simulink model "lab_1_n_4"  (R2021b)
settings: Solver=VariableStepAuto  StartTime=0.0  StopTime=100.0  RelTol=1e-3
libraries: simulink x1
settings Model: Creator=peter  LastModifiedBy=peter

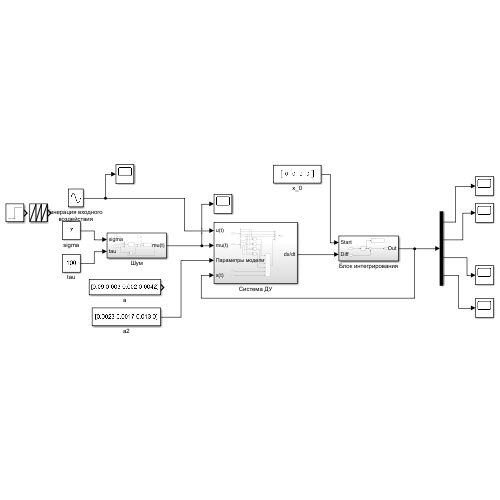
[thumbnail: Simulink's stored preview of the top-level diagram]
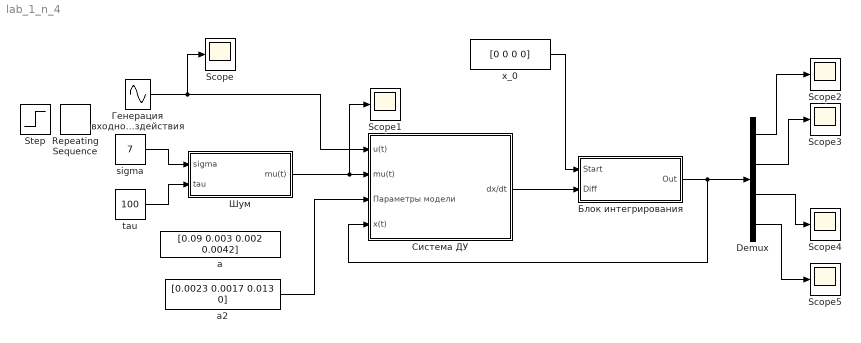
== system lab_1_n_4 ==
  Demux : Demux
  Repeating Sequence : simulink/Sources/Repeating Sequence  rep_seq_t=[0 2]  rep_seq_y=[0 2]
  Scope{,1..5} (6 alike) : Scope
  Step : Step  Time=10  SampleTime=0
  a : Constant  Value=[0.09 0.003 0.002 0.0042]
  a2 : Constant  Value=[0.0023 0.0017 0.013 0]
  sigma : Constant  Value=7
  tau : Constant  Value=100
  x_0 : Constant  Value=[0 0 0 0]
  Блок интегрирования : Subsystem
  Генерация входного воздействия : Sin  Frequency=0.05  SampleTime=0
  Система ДУ : Subsystem
  Шум : Subsystem
  wires:
  Demux/1 -> Scope2/1
  Demux/2 -> Scope3/1
  Demux/4 -> Scope5/1
  Demux/3 -> Scope4/1
  Блок интегрирования/1(Out) -> Система ДУ/4(x(t)), Demux/1
  x_0/1 -> Блок интегрирования/1(Start)
  Система ДУ/1(dx/dt) -> Блок интегрирования/2(Diff)
  Шум/1(mu(t)) -> Scope1/1, Система ДУ/2(mu(t))
  tau/1 -> Шум/2(tau)
  sigma/1 -> Шум/1(sigma)
  Генерация входного воздействия/1 -> Scope/1, Система ДУ/1(u(t))
  a2/1 -> Система ДУ/3(Параметры модели)

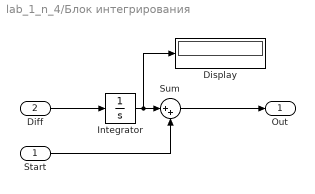
== system lab_1_n_4/Блок интегрирования ==
  Start : Inport
  Diff : Inport  Port=2
  Display : Display
  Integrator : Integrator
  Sum : Sum  Inputs=|++
  Out : Outport
  wires:
  Diff/1 -> Integrator/1
  Sum/1 -> Out/1
  Integrator/1 -> Display/1, Sum/1
  Start/1 -> Sum/2

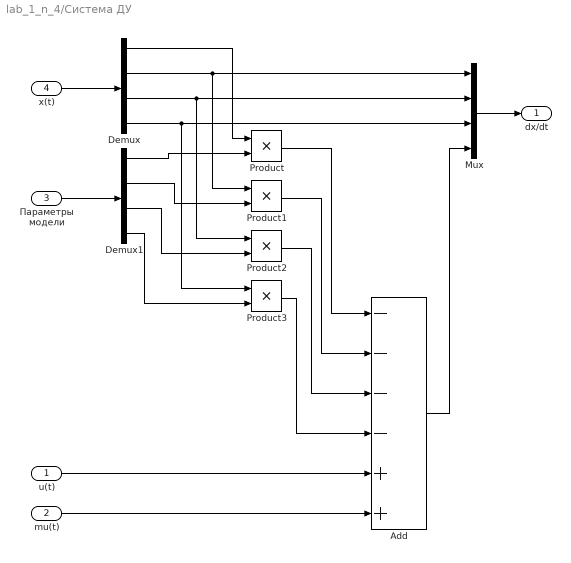
== system lab_1_n_4/Система ДУ ==
  u(t) : Inport
  mu(t) : Inport  Port=2
  Параметры модели : Inport  Port=3
  x(t) : Inport  Port=4
  Add : Sum  Inputs=----++
  Demux : Demux
  Demux1 : Demux
  Mux : Mux
  Product{,1..3} (4 alike) : Product
  dx/dt : Outport
  wires:
  x(t)/1 -> Demux/1
  Параметры модели/1 -> Demux1/1
  Mux/1 -> dx/dt/1
  Demux1/1 -> Product/2
  Demux1/2 -> Product1/2
  Demux1/3 -> Product2/2
  Demux/1 -> Product/1
  Demux/2 -> Product1/1, Mux/1
  Demux/3 -> Product2/1, Mux/2
  Product/1 -> Add/1
  Product1/1 -> Add/2
  Product2/1 -> Add/3
  Demux1/4 -> Product3/2
  Add/1 -> Mux/4
  Demux/4 -> Product3/1, Mux/3
  u(t)/1 -> Add/5
  Product3/1 -> Add/4
  mu(t)/1 -> Add/6

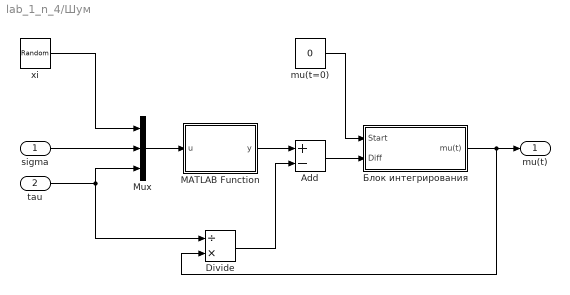
== system lab_1_n_4/Шум ==
  sigma : Inport
  tau : Inport  Port=2
  Add : Sum  Inputs=+-
  Divide : Product  Inputs=/*
  MATLAB Function : MATLAB Function  TreatAsAtomicUnit=on
  Mux : Mux  Inputs=3
  mu(t=0) : Constant  Value=0
  xi : RandomNumber  SampleTime=0.1
  Блок интегрирования : Subsystem
  mu(t) : Outport
  wires:
  mu(t=0)/1 -> Блок интегрирования/1(Start)
  Блок интегрирования/1(mu(t)) -> Divide/2, mu(t)/1
  xi/1 -> Mux/1
  sigma/1 -> Mux/2
  tau/1 -> Divide/1, Mux/3
  Add/1 -> Блок интегрирования/2(Diff)
  Divide/1 -> Add/2
  MATLAB Function/1(y) -> Add/1
  Mux/1 -> MATLAB Function/1(u)

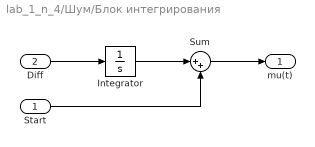
== system lab_1_n_4/Шум/Блок интегрирования ==
  Start : Inport
  Diff : Inport  Port=2
  Integrator : Integrator
  Sum : Sum  Inputs=|++
  mu(t) : Outport
  wires:
  Integrator/1 -> Sum/1
  Sum/1 -> mu(t)/1
  Diff/1 -> Integrator/1
  Start/1 -> Sum/2

== matlab function lab_1_n_4/Шум/MATLAB Function ==
  data: u input; y output
function y = fcn(u)
    xi=u(1);
    sigma=u(2);
    tau=u(3);
    alpha=1/tau;
    k_f=sigma*sqrt(2*alpha);
y = k_f*xi;
